simulink library "zynq_API"  (R2017a)
settings: Solver=VariableStepAuto  StartTime=0.0  StopTime=10.0  RelTol=1e-3
settings Model: Creator=htkim  LastModifiedBy=htkim

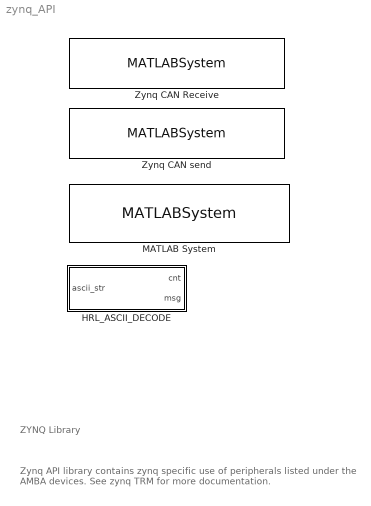
== system zynq_API ==
  note: ZYNQ Library
  note: Zynq API library contains zynq specific use
      | of peripherals listed under the AMBA devices.
      | See zynq TRM for more documentation.
  HRL_ASCII_DECODE : Subsystem  TreatAsAtomicUnit=on
  MATLAB System : MATLABSystem  System=zynq_RS232.txrx  BaudRate=19200  MessageLength=16
      mask Type: zynq_RS232.txrx
      mask Display:
      | disp('Zynq RS232');
      | port_label('input',1,'Tx Data');
      | port_label('input',2,'Tx Length');
      | port_label('output',1,'Rx Data');
      | port_label('output',2,'Data length');
  Zynq CAN Receive : MATLABSystem  System=zynq_CAN.recv  CANDev=can0  Timeout=Inf  FilterEnable=on  FilterIDs=0  FilterMasks=0
      mask Type: zynq_CAN.recv
      mask Display:
      | disp('CAN Receive');
      | port_label('output',1,'Status');
      | port_label('output',2,'ID');
      | port_label('output',3,'Data');
      | port_label('output',4,'Timestamp');
  Zynq CAN send : MATLABSystem  System=zynq_CAN.send  CANID=0  CANDev=can0
      mask Type: zynq_CAN.send
      mask Display:
      | disp('CAN Send');
      | port_label('input',1,'Data');
      | port_label('output',1,'Status');

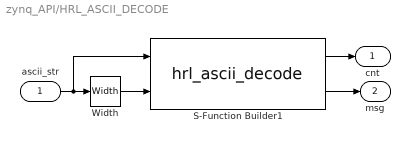
== system zynq_API/HRL_ASCII_DECODE ==
  ascii_str : Inport
  S-Function Builder1 : S-Function  InitFcn=try, set_param(gcb,'FunctionName','hrl_ascii_decode'), end  FunctionName=hrl_ascii_decode  SFunctionModules=hrl_ascii_decode_wrapper  SFunctionDeploymentMode=off  EnableBusSupport=off  mask(S-Function Builder){}
      mask help: Simulink:masks:SFunctionBuilder_MD
      mask init:
      | val = [[.9  0.75 0.75 1 1 .9 .9 1]',[1 1 0.75 0.75 .9 .9 1 .9]'];try , sys = get_param(gcb,'SfunBuilderFcnName');if isempty(sys), sys = get_param(gcb,'FunctionName'); end,catch, sys = get_param(gcb,'FunctionName'); end
      settings: CopyFcn=set_param(gcbh,'LinkStatus','none')  PreSaveFcn=try, set_param(gcb,'FunctionName','hrl_ascii_decode'), end  OpenFcn=sfunctionwizard(gcbh)
      mask Display: plot(val(:,1),val(:,2)),disp(sys), port_label('input',1,'str'), port_label('input',2,'len'), port_label('output',1,'cnt'), port_label('output',2,'msg')
  Width : Width
  cnt : Outport
  msg : Outport  Port=2
  wires:
  ascii_str/1 -> S-Function Builder1/1, Width/1
  Width/1 -> S-Function Builder1/2
  S-Function Builder1/2 -> msg/1
  S-Function Builder1/1 -> cnt/1
